simulink subsystem "PVInverterGFL"  (R2023a)
settings: Solver=VariableStepAuto  StartTime=0.0  StopTime=10.0  RelTol=1e-3
model mask{c=PVInverter.C, c_unit=F, g=0, g_unit=1/Ohm, vc_priority=None, vc_specify=on, vc=PVInverter.Vdc, vc_unit=V, Pfixed=1, Pfixed_unit=W, L=PVInverter.L, L_unit=H, R=1e-3, R_unit=Ohm, VRated=Base.KV_base_new, SRated=Base.MVA_base_new}
  mask prompts: c "Capacitance"; g "Parallel conductance"; vc_priority "Initial voltage priority"; vc_specify "Initial voltage"; vc "Initial vc"; Pfixed "Fixed power loss"; L "Filter inductance"; R "Filter resistance"; VRated "Nominal voltage (phase-to-phase RMS in V)"; SRated "Nominal power (in V*A)"
undefined symbols (not defined in the file): Ts
libraries: fl_lib x4, nesl_utility x4, ee_lib x3, spsLeadLagFilterLib x2
settings Model: Creator=rajarshd  LastModifiedBy=rajarshd

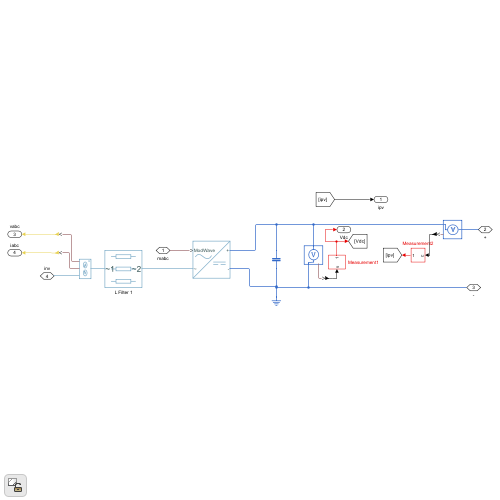
[thumbnail: Simulink's stored preview of the top-level diagram]
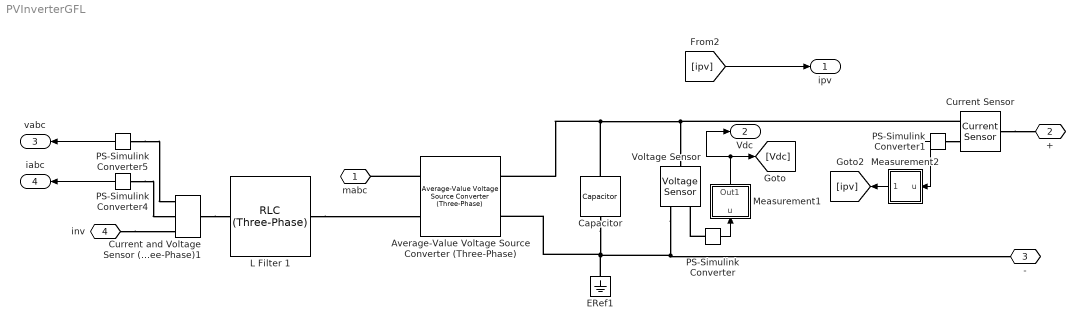
== system PVInverterGFL ==
  Average-Value Voltage Source Converter (Three-Phase) : ee_lib/Semiconductors & Converters/Converters/Average-Value Voltage Source Converter (Three-Phase)  port_option=ee.enum.threePhasePort.composite  frequency_option=ee.enum.converters.frequency.variable  FRated=60 Hz  losses_parameterization=ee.enum.converters.losses.fixed  Pfixed=Pfixed W  ks=0.01  kc1=1.7 V  kc2=0.01 Ohm  Ploss_vect=[100, 800, 1870, 3250, 4900] W  Irms_vect=[10, 100, 200, 300, 400] A  Vdc_nom=300 V  thermal_mass=30000 J/K  temperature_specify=off  temperature_priority=High  temperature=298.15 K  temperature_nominal_specify=off  temperature_nominal_unit=K  temperature_nominal_value=1
      settings: InternalSimscapePortConfiguration="{\"Bottom\":[],\"Left\":[{\"id\":\"ModWave\",\"label\":\"ModWave\",\"type\":\"input\"},{\"id\":\"N\",\"label\":\"~\",\"type\":\"foundation.electrical.three_phase\"}],\"Right\":[{\"id\":\"p\",\"label\":\"+\",\"type\":\"foundation.electrical.electrical\"},{\"id\":\"n\",\"label\":\"-\",\"type\":\"foundation.electrical.electrical\"}],\"Top\":[]}"
  Capacitor : fl_lib/Electrical/Electrical Elements/Capacitor  c=c F  r=1e-6 Ohm  g=g 1/Ohm  i_specify=off  i_priority=None  i=0 A  i_nominal_specify=off  i_nominal_unit=A  i_nominal_value=1  v_specify=off  v_priority=None  v=6560*.5 V  v_nominal_specify=off  v_nominal_unit=V  v_nominal_value=1  vc_specify=on  vc_priority=None  vc=vc V  vc_nominal_specify=off  vc_nominal_unit=V  vc_nominal_value=1
  Current Sensor : fl_lib/Electrical/Electrical Sensors/Current Sensor
  Current and Voltage Sensor (Three-Phase)1 : ee_lib/Sensors & Transducers/Current and Voltage Sensor (Three-Phase)  vMeasurementType=ee.enum.vmeasurement.lg  outputUnit=ee.enum.unit.pu  SRated=SRated A*V  VRated=VRated V  I_specify=off  I_priority=None  I=[0, 0, 0] A  I_nominal_specify=off  I_nominal_unit=A  I_nominal_value=1  V_specify=off  V_priority=None  V=[0, 0, 0] V  V_nominal_specify=off  V_nominal_unit=V  V_nominal_value=1
      settings: InternalSimscapePortConfiguration="{\"Bottom\":[],\"Left\":[{\"id\":\"N1\",\"label\":\"~1\",\"type\":\"foundation.electrical.three_phase\"}],\"Right\":[{\"id\":\"V_output\",\"label\":\"V\",\"type\":\"output\"},{\"id\":\"I_output\",\"label\":\"I\",\"type\":\"output\"},{\"id\":\"N2\",\"label\":\"~2\",\"type\":\"foundation.electrical.three_phase\"}],\"Top\":[]}"
  ERef1 : fl_lib/Electrical/Electrical Elements/Electrical Reference
  L Filter 1 : ee_lib/Passive/RLC Assemblies/RLC (Three-Phase)  component_structure=ee.enum.rlc.structure.L  R=1e-3 Ohm  L=L H  C=1e-6 F  R_parasitic=0 Ohm  G_parasitic=0 1/Ohm  IL_specify=off  IL_priority=High  IL=[0, 0, 0] A  IL_nominal_specify=off  IL_nominal_unit=A  IL_nominal_value=1  VC_specify=off  VC_priority=High  VC=[0, 0, 0] V  VC_nominal_specify=off  VC_nominal_unit=V  VC_nominal_value=1
      settings: InternalSimscapePortConfiguration="{\"Bottom\":[],\"Left\":[{\"id\":\"N1\",\"label\":\"~1\",\"type\":\"foundation.electrical.three_phase\"}],\"Right\":[{\"id\":\"N2\",\"label\":\"~2\",\"type\":\"foundation.electrical.three_phase\"}],\"Top\":[]}"
  Measurement1 : Subsystem
  Measurement2 : Subsystem
  PS-Simulink Converter{,1,4..5} (4 alike) : nesl_utility/PS-Simulink Converter  PhysicalDomain=network_engine_domain  SubClassName=ps_output  LeftPortType=input  RightPortType=output  PseudoPeriodic=off  Frequencies=[]  VectorFormat=inherit  Unit=inherit  AffineConversion=off
  Voltage Sensor : fl_lib/Electrical/Electrical Sensors/Voltage Sensor
  mabc : PMIOPort  Side=Left
  + : PMIOPort  Port=2  Side=Left
  - : PMIOPort  Port=3  Side=Left
  inv : PMIOPort  Port=4  Side=Right
  ipv : Outport
  Vdc : Outport  Port=2
  vabc : Outport  Port=3
  iabc : Outport  Port=4
  wires:
  Measurement1/1(Out1) -> [Vdc], Vdc/1
  PS-Simulink Converter/1 -> Measurement1/1(u)
  PS-Simulink Converter1/1 -> Measurement2/1(u)
  Measurement2/1(Out1) -> [ipv]
  [ipv] -> ipv/1
  PS-Simulink Converter5/1 -> vabc/1
  PS-Simulink Converter4/1 -> iabc/1
  connections:
  ERef1/LConn1 -- -/RConn1 -- Voltage Sensor/RConn2 -- Average-Value Voltage Source Converter (Three-Phase)/RConn2 -- Capacitor/RConn1
  Capacitor/LConn1 -- Average-Value Voltage Source Converter (Three-Phase)/RConn1 -- Voltage Sensor/LConn1 -- Current Sensor/RConn2
  PS-Simulink Converter/LConn1 -- Voltage Sensor/RConn1
  PS-Simulink Converter1/LConn1 -- Current Sensor/RConn1
  L Filter 1/RConn1 -- Average-Value Voltage Source Converter (Three-Phase)/LConn2
  Current Sensor/LConn1 -- +/RConn1
  Average-Value Voltage Source Converter (Three-Phase)/LConn1 -- mabc/RConn1
  PS-Simulink Converter4/LConn1 -- Current and Voltage Sensor (Three-Phase)1/RConn2
  PS-Simulink Converter5/LConn1 -- Current and Voltage Sensor (Three-Phase)1/RConn1
  Current and Voltage Sensor (Three-Phase)1/LConn1 -- L Filter 1/LConn1
  inv/RConn1 -- Current and Voltage Sensor (Three-Phase)1/RConn3

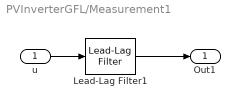
== system PVInverterGFL/Measurement1 ==
  u : Inport
  Lead-Lag Filter1 : spsLeadLagFilterLib/Lead-Lag Filter  T1=0  T2=Grid.sensor_time  Vdc_Init=0  Ts=Ts
  Out1 : Outport
  wires:
  u/1 -> Lead-Lag Filter1/1
  Lead-Lag Filter1/1 -> Out1/1

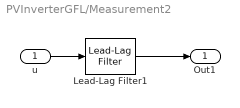
== system PVInverterGFL/Measurement2 ==
  u : Inport
  Lead-Lag Filter1 : spsLeadLagFilterLib/Lead-Lag Filter  T1=0  T2=Grid.sensor_time  Vdc_Init=0  Ts=Ts
  Out1 : Outport
  wires:
  u/1 -> Lead-Lag Filter1/1
  Lead-Lag Filter1/1 -> Out1/1
